simulink model "es2_comando"  (R2014a)
settings: Solver=ode45  StartTime=0.0  StopTime=5  RelTol=1e-3
values from neighbouring files (symbols this model uses):
  Kr = 2    [es2.m]
libraries: cstblocks x2
settings Model: Creator=HP  LastModifiedBy=HP

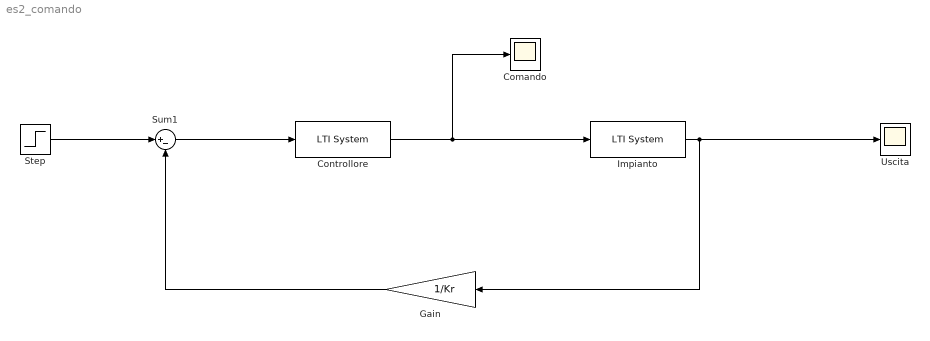
== system es2_comando ==
  "Comando " : Scope
      settings: SaveName=ScopeData2
  Controllore : cstblocks/LTI System  sys=C  IC=[]
  Gain : Gain  Gain=1/Kr
  Impianto : cstblocks/LTI System  sys=F  IC=[]
  Step : Step  Time=0  SampleTime=0
  Sum1 : Sum  Inputs=|+-
  Uscita : Scope
  wires:
  Sum1/1 -> Controllore/1
  Gain/1 -> Sum1/2
  Step/1 -> Sum1/1
  Impianto/1 -> Uscita/1, Gain/1
  Controllore/1 -> Impianto/1, "Comando "/1
